simulink model "Cooperative_Quad_09_VelEst_02"  (R2017b)
settings: Solver=ode45  StartTime=0.0  StopTime=120  RelTol=1e-3  EnableMultiTasking=on
InitFcn:
  | Const_Vel_Est_02
values from neighbouring files (symbols this model uses):
  alpha = 1.0e-5    (= 1e-05)    [Cons_AMFC_Quad_New_01.m]    (also in Const_Vel_Est_02.m = 0.1; constant_Rev01_4Agents_10.m = 0.1; constant_Rev01_4Agents_9.m = 0.1)
  alpha_Slid = 0.01    [Cons_AMFC_Quad_New_01.m]    (also in Const_Vel_Est_02.m)
  AN = [     0 1 0 0 ... (first row only)    [Const_Vel_Est_02.m]    (also in constant_Rev01_4Agents_10.m; constant_Rev01_4Agents_9.m)
  B = 1e+0*eye(n)    [Cons_AMFC_Quad_New_01.m]    (also in Const_Vel_Est_02.m = 1e0*eye(n); constant_Rev01_4Agents_10.m = 1e0*eye(n); constant_Rev01_4Agents_9.m = 1e0*eye(n))
  BBT_inv = ((B'*B)^(-1))*B'    [Cons_AMFC_Quad_New_01.m]    (also in Const_Vel_Est_02.m; constant_Rev01_4Agents_10.m; constant_Rev01_4Agents_9.m)
  BN = [     1 0 0 0 ... (first row only)    [Const_Vel_Est_02.m]    (also in constant_Rev01_4Agents_10.m; constant_Rev01_4Agents_9.m)
  epsilon_struct = struct('data',epsilon_InitVal)    [Const_Vel_Est_02.m]    (also in constant_Rev01_4Agents_10.m; constant_Rev01_4Agents_9.m)
  g = 9.81    [Const_Vel_Est_02.m]    (also in Swing2d_01_const.m; constant_Rev01_4Agents_10.m; constant_Rev01_4Agents_9.m)
  gamma_0 = 1e-0*diag([1e-3*ones(3,1);1e-0*ones(3,1)])    [Cons_AMFC_Quad_New_01.m]    (also in Const_Vel_Est_02.m = 1e-1*diag([1e-3*ones(3,1);1e-0*ones(3,1)]); constant_Rev01_4Agents_10.m = 1e+1*diag([1e-3*ones(3,1);1e-0*ones(3,1)]); constant_Rev01_4Agents_9.m = 1e+1*diag([1e-3*ones(6,1);1e-0*ones(6,1)]))
  gamma_1 = 1e+2*diag([1e-3*ones(3,1);1e-0*ones(3,1)])    [Cons_AMFC_Quad_New_01.m]    (also in Const_Vel_Est_02.m; constant_Rev01_4Agents_10.m = 1e+3*diag([1e-3*ones(3,1);1e0*ones(3,1)]); constant_Rev01_4Agents_9.m = 1e+3*diag([1e-3*ones(6,1);1e0*ones(6,1)]))
  H = L + BN    [Const_Vel_Est_02.m]    (also in constant_Rev01_4Agents_10.m; constant_Rev01_4Agents_9.m)
  J = 1.2416e-3 * diag([1 1 2])    [Cons_AMFC_Quad_New_01.m]    (also in Const_Vel_Est_02.m = 1.2416e-3 * diag([1 1 2],0); constant_Rev01_4Agents_10.m = 1.2416e-3 * diag([1 1 2],0); constant_Rev01_4Agents_9.m = 1.2416e-3 * diag([1 1 2],0))
  k1 = 10    [Cons_AMFC_Quad_New_01.m]    (also in Const_Vel_Est_02.m = 1; constant_Rev01_4Agents_10.m = 1; constant_Rev01_4Agents_9.m = 1)
  k1o = 1000    [Cons_AMFC_Quad_New_01.m]    (also in Const_Vel_Est_02.m)
  k2 = 0.1    [Cons_AMFC_Quad_New_01.m]    (also in Const_Vel_Est_02.m; constant_Rev01_4Agents_10.m = 1; constant_Rev01_4Agents_9.m = 1)
  k2o = 100    [Cons_AMFC_Quad_New_01.m]    (also in Const_Vel_Est_02.m)
  Ka = 0.01    [Cons_AMFC_Quad_New_01.m]    (also in Const_Vel_Est_02.m; constant_Rev01_4Agents_10.m; constant_Rev01_4Agents_9.m)
  Kd = 0.01    [Cons_AMFC_Quad_New_01.m]    (also in Const_Vel_Est_02.m; constant_Rev01_4Agents_10.m; constant_Rev01_4Agents_9.m)
  Kf = 1.0e-5    (= 1e-05)    [Cons_AMFC_Quad_New_01.m]    (also in Const_Vel_Est_02.m; constant_Rev01_4Agents_10.m; constant_Rev01_4Agents_9.m)
  Kt = 0.0435 * Kf    (= 4.35e-07)    [Cons_AMFC_Quad_New_01.m]    (also in Const_Vel_Est_02.m = 1e-07; constant_Rev01_4Agents_10.m = 1e-07; constant_Rev01_4Agents_9.m = 1e-07)
  Lq = 0.2    [Const_Vel_Est_02.m]    (also in constant_Rev01_4Agents_10.m; constant_Rev01_4Agents_9.m)
  m = 6    [Cons_AMFC_Quad_New_01.m]    (also in Const_Vel_Est_02.m; Swing2d_01_const.m = 1)
  M = 2.95    [Cons_AMFC_Quad_New_01.m]    (also in Const_Vel_Est_02.m = 2; constant_Rev01_4Agents_10.m = 2; constant_Rev01_4Agents_9.m = 2)
  Mb_P = Mb_val_P*ones(np,1)    [Const_Vel_Est_02.m]
  Mb_V = Mb_val_V*ones(np,1)    [Const_Vel_Est_02.m]
  Mu_P = 10    [Const_Vel_Est_02.m]
  Mu_V = 10    [Const_Vel_Est_02.m]
  n = 6    [Cons_AMFC_Quad_New_01.m]    (also in Const_Vel_Est_02.m; constant_Rev01_4Agents_10.m; constant_Rev01_4Agents_9.m = 12)
  N = 4    [Const_Vel_Est_02.m]    (also in constant_Rev01_4Agents_10.m; constant_Rev01_4Agents_9.m)
  n0 = 3    [Const_Vel_Est_02.m]    (also in constant_Rev01_4Agents_10.m; constant_Rev01_4Agents_9.m)
  np = 2    [Const_Vel_Est_02.m]
  Observer_Gain = 100    [Const_Vel_Est_02.m]    (also in constant_Rev01_4Agents_10.m; constant_Rev01_4Agents_9.m)
  Observer_Gain1 = 100    [Const_Vel_Est_02.m]    (also in constant_Rev01_4Agents_10.m = 10; constant_Rev01_4Agents_9.m = 10)
  Q = 1e-1*eye(n)    [Cons_AMFC_Quad_New_01.m]    (also in Const_Vel_Est_02.m = 1e-2*eye(n); constant_Rev01_4Agents_10.m = 1e-3*eye(n); constant_Rev01_4Agents_9.m = 1e-3*eye(n))
  R = 1e+0*eye(m)    [Cons_AMFC_Quad_New_01.m]    (also in Const_Vel_Est_02.m = 1e-0*eye(n); constant_Rev01_4Agents_10.m = 1e-0*eye(n); constant_Rev01_4Agents_9.m = 1e-0*eye(n))
  rho_0 = 1e-1    (= 0.1)    [Cons_AMFC_Quad_New_01.m]    (also in Const_Vel_Est_02.m; constant_Rev01_4Agents_10.m = 10; constant_Rev01_4Agents_9.m = 10)
  rho_1 = 1e-0    (= 1)    [Cons_AMFC_Quad_New_01.m]    (also in Const_Vel_Est_02.m; constant_Rev01_4Agents_10.m = 0.1; constant_Rev01_4Agents_9.m = 0.1)
  T_struct = struct('data',T_InitVal)    [Const_Vel_Est_02.m]    (also in constant_Rev01_4Agents_10.m; constant_Rev01_4Agents_9.m)
  U_dot0_M = U_dot0_m*ones(n0,1)    [Const_Vel_Est_02.m]    (also in constant_Rev01_4Agents_10.m; constant_Rev01_4Agents_9.m)
  Upsilon_M = Upsilon_m*ones(n0,1)    [Const_Vel_Est_02.m]    (also in constant_Rev01_4Agents_10.m; constant_Rev01_4Agents_9.m)
undefined symbols (not defined in the file or in its folder): sigbuilder_block
(part 5 of 5)

== matlab function Cooperative_Quad_09_VelEst_02/Agent #4/Decenteralized Cooperaive Controller #4/Ali-4/Translational-4/Differentiator/Sliding differentiator1 ==
  data: Du1 output; e input; n parameter; k2 parameter
function Du1 = fcn(e,n,k2)

a=k2;

ABS = zeros(n,1);
for i=1:n
    if e(i)>0
        ABS(i) = e(i);
    else
        ABS(i) = -e(i);
    end
end
SGN = e ./ (ABS + 0.01);

Du1 = - a*SGN;

end

== matlab function Cooperative_Quad_09_VelEst_02/Agent #4/Decenteralized Cooperaive Controller #4/Ali-4/Translational-4/g-Estimator ==
  data: sigma input; g_hat input; P input; rho_1 parameter; gamma_1 parameter; Dg_hat output
function Dg_hat = fcn(sigma,g_hat,P,rho_1,gamma_1)

Dg_hat = - gamma_1 * P * sigma - rho_1 * gamma_1 * g_hat;

end

== matlab function Cooperative_Quad_09_VelEst_02/Agent #4/Decenteralized Cooperaive Controller #4/Ali-4/Translational-4/main ==
  data: sigma input; zeta input; u output; Dy_d input; R parameter; P input; a_hat input; B parameter; g_hat input; x input; Q parameter; BBT_inv parameter; n parameter
function u = fcn(sigma,zeta,Dy_d,R,P,a_hat,B,g_hat,x,Q,BBT_inv,n)

u1 = (1/2) * R * B' * P * sigma;
u2 = BBT_inv * (Dy_d - a_hat*x + (eye(n) + 2*(((P)^(-1)*Q)) + a_hat)*sigma - g_hat - zeta) - (3/4) * R * B' * P * sigma;

u = u1 + u2;

end

== matlab function Cooperative_Quad_09_VelEst_02/Agent #4/Decenteralized Cooperaive Controller #4/Ali-4/Translational-4/variable change ==
  data: X input; Xd input; x_mod output; u input; xd_mod output; e_mod output
function [x_mod,xd_mod,e_mod] = fcn(X,Xd,u)

x_mod = [X(1:3);X(7:9)];

xd_mod = [Xd;u(1:3)];

e_mod = xd_mod - x_mod;


end

== matlab function Cooperative_Quad_09_VelEst_02/Agent #4/Decenteralized Cooperaive Controller #4/Computing xd-4  ==
  data: q_i input; T_i input; xd output; Agent_Num input
function xd = fcn(q_i,T_i,Agent_Num)

xd = q_i + T_i(1,:)' + T_i(Agent_Num+1,:)';

end

== matlab function Cooperative_Quad_09_VelEst_02/Agent #4/Decenteralized Cooperaive Controller #4/Cooperative Observers for X-4/Differentiator2/Sliding differentiator ==
  data: u output; u1 input; e input; k1o parameter; alpha_Slid parameter
function u = fcn(u1,e,k1o,alpha_Slid)

b=k1o;

ABS = abs(e);
SGN = e ./ (ABS + alpha_Slid);
u = u1 - b*((ABS.^0.5).*SGN); 

end

== matlab function Cooperative_Quad_09_VelEst_02/Agent #4/Decenteralized Cooperaive Controller #4/Cooperative Observers for X-4/Differentiator2/Sliding differentiator1 ==
  data: Du1 output; e input; k2o parameter; alpha_Slid parameter
function Du1 = fcn(e,k2o,alpha_Slid)

a=k2o;

ABS = abs(e);
SGN = e ./ (ABS + alpha_Slid);
Du1 = - a*SGN;

end

== matlab function Cooperative_Quad_09_VelEst_02/Agent #4/Decenteralized Cooperaive Controller #4/Cooperative Observers for X-4/MATLAB Function ==
  data: X_inp input; X_est output; P_est_XY input; Pos_local_Z input; V_est_XY input; V_local_Z input
function X_est = fcn(X_inp,P_est_XY,Pos_local_Z,V_est_XY,V_local_Z)

X_est = [P_est_XY;Pos_local_Z;X_inp(4:6);V_est_XY;V_local_Z;X_inp(10:12)];

end

== matlab function Cooperative_Quad_09_VelEst_02/Agent #4/Decenteralized Cooperaive Controller #4/Cooperative Observers for X-4/Pos observer-4 ==
  data: P_hat input; tau input; P0 input; P_rel_local input; P_rel0_local input; AN parameter; BN parameter; H parameter; DP_hat_local output; np parameter; N parameter; Num input; Mu_P parameter; Mb_P parameter; tau_i output; alpha parameter
function [DP_hat_local,tau_i] = fcn(P_hat,tau,P0,P_rel_local,P_rel0_local,AN,BN,H,np,N,Num,Mu_P,Mb_P,alpha)

P_hat_in = zeros(np,N);
P_rel_local_in = zeros(np,N);
tau_in = zeros(np,N);
for i=1:N
    P_hat_in(:,i) = P_hat((i-1)*np+1:(i*np),1); 
    P_rel_local_in(:,i) = P_rel_local((i-1)*np+1:(i*np),1); 
    tau_in(:,i) = tau((i-1)*np+1:(i*np),1);
end

e = BN(Num,Num)*(P_hat_in(:,Num) - (P0 + P_rel0_local));
Vec = zeros(np,1);
for i=1:N
    e = e + ( AN(Num,i)*(P_hat_in(:,Num) - (P_hat_in(:,i) + P_rel_local_in(:,i))) ); 
    Vec = Vec + ( H(Num,i)*tau_in(:,i) );    
end

SGN_vec = Vec./(abs(Vec)+alpha);
SGN = diag(SGN_vec);    

DP_hat_local = - ( Mu_P*e ) - ( SGN*Mb_P );
tau_i = e;

end

== matlab function Cooperative_Quad_09_VelEst_02/Agent #4/Decenteralized Cooperaive Controller #4/Cooperative Observers for X-4/Vel observer-4 ==
  data: P_hat input; tau input; P0 input; P_rel_local input; P_rel0_local input; AN parameter; BN parameter; H parameter; DP_hat_local output; np parameter; N parameter; Num input; Mu_V parameter; Mb_V parameter; tau_i output; alpha parameter
function [DP_hat_local,tau_i] = fcn(P_hat,tau,P0,P_rel_local,P_rel0_local,AN,BN,H,np,N,Num,Mu_V,Mb_V,alpha)

P_hat_in = zeros(np,N);
P_rel_local_in = zeros(np,N);
tau_in = zeros(np,N);
for i=1:N
    P_hat_in(:,i) = P_hat((i-1)*np+1:(i*np),1); 
    P_rel_local_in(:,i) = P_rel_local((i-1)*np+1:(i*np),1); 
    tau_in(:,i) = tau((i-1)*np+1:(i*np),1);
end

e = BN(Num,Num)*(P_hat_in(:,Num) - (P0 + P_rel0_local));
Vec = zeros(np,1);
for i=1:N
    e = e + ( AN(Num,i)*(P_hat_in(:,Num) - (P_hat_in(:,i) + P_rel_local_in(:,i))) ); 
    Vec = Vec + ( H(Num,i)*tau_in(:,i) );    
end

SGN_vec = Vec./(abs(Vec)+alpha);
SGN = diag(SGN_vec);    

DP_hat_local = - ( Mu_V*e ) - ( SGN*Mb_V );
tau_i = e;

end

== matlab function Cooperative_Quad_09_VelEst_02/Agent #4/Decenteralized Cooperaive Controller #4/Cooperative Observers for Xd-4/Observer T#4 ==
  data: T_struct parameter; T input; DT_i output; epsilon input; epsilon_struct parameter; H parameter; BN parameter; AN parameter; T_i input; chi input; Upsilon_M parameter; epsilon_i output; N parameter; n0 parameter; Agent_Num input; Observer_Gain1 parameter; alpha parameter
function [DT_i,epsilon_i] = fcn(T_struct,T,epsilon,epsilon_struct,H,BN,AN,T_i,chi,Upsilon_M,N,n0,...
    Agent_Num,Observer_Gain1,alpha)

T_struct(1).data = T.t1;
T_struct(2).data = T.t2;
T_struct(3).data = T.t3;
T_struct(4).data = T.t4;

epsilon_struct(1).data = epsilon.eps1;
epsilon_struct(2).data = epsilon.eps2;
epsilon_struct(3).data = epsilon.eps3;
epsilon_struct(4).data = epsilon.eps4;

epsilon_i = + BN(Agent_Num,Agent_Num)*(T_i - chi);
Sum2 = zeros(N+1,n0);
for i=1:N
    epsilon_i = epsilon_i + ( AN(Agent_Num,i) * (T_i - T_struct(i).data) );  
    Sum2 = Sum2 + ( H(i,Agent_Num) * epsilon_struct(i).data );
end

Sum21 = abs(Sum2) + alpha;
SGN2 = Sum2./Sum21;

DT_i = -Observer_Gain1*epsilon_i - SGN2*diag(Upsilon_M);

end

== matlab function Cooperative_Quad_09_VelEst_02/Agent #4/Decenteralized Cooperaive Controller #4/Cooperative Observers for Xd-4/Observer q#4 ==
  data: q input; Dq_i output; tau input; H parameter; BN parameter; AN parameter; q_i input; u0 input; U_dot0_M parameter; tau_i output; N parameter; Agent_Num input; Observer_Gain parameter; n0 parameter; alpha parameter
function [Dq_i,tau_i] = fcn(q,tau,H,BN,AN,q_i,u0,U_dot0_M,N,Agent_Num,Observer_Gain,n0,alpha)

tau_i = + BN(Agent_Num,Agent_Num)*(q_i - u0);
Sum2 = zeros(n0,1);
for i=1:N
    tau_i = tau_i + ( AN(Agent_Num,i) * (q_i - q(((i-1)*n0+1):n0*i)) );  
    Sum2 = Sum2 + ( H(i,Agent_Num) * tau(((i-1)*n0+1):n0*i) );
end

Sum21 = abs(Sum2) + alpha;
SGN2 = Sum2./Sum21;

Dq_i = -Observer_Gain*tau_i - diag(SGN2)*U_dot0_M;

end

== matlab function Cooperative_Quad_09_VelEst_02/Agent #4/Plant #4/MATLAB Function ==
  data: X input; u1 input; u2 input; u3 input; u4 input; t input; DX output; Kf parameter; Kt parameter; Kd parameter; Ka parameter; M parameter; J parameter; Lq parameter; g parameter; Pos_XY output; Pos_Z output; Vel_XY output; Acc_XY output
function [DX,Pos_XY,Pos_Z,Vel_XY,Acc_XY] = fcn(X,u1,u2,u3,u4,t,Kf,Kt,Kd,Ka,M,J,Lq,g)

F1 = Kf * u1^2;
F2 = Kf * u2^2;
F3 = Kf * u3^2;
F4 = Kf * u4^2;
 
FT = F1 + F2 + F3 + F4;

T1 = Kt * u1^2;
T2 = Kt * u2^2;
T3 = Kt * u3^2;
T4 = Kt * u4^2;

phi = X(4);
theta = X(5);
psi = X(6);

Rq = [cos(psi)*cos(theta) -sin(psi)*cos(phi)+cos(psi)*sin(theta)*sin(phi) sin(psi)*sin(phi)+cos(psi)*sin(theta)*cos(phi);
    sin(psi)*cos(theta) cos(psi)*cos(phi)+sin(psi)*sin(theta)*sin(phi) -cos(psi)*sin(phi)+sin(psi)*sin(theta)*cos(phi);
    -sin(theta) cos(theta)*sin(phi) cos(theta)*cos(phi)]; 

R_omega = [1 0 -sin(theta);
    0 cos(phi) cos(theta)*sin(phi);
    0 -sin(phi) cos(theta)*cos(phi)];

EXT_PRD = External_Product3(X(10:12),(J*X(10:12)));

DP = X(7:9);
DPHI = R_omega^(-1) * X(10:12); 
Dv = (1/M)*(Rq*[0;0;FT] - Kd*X(7:9) - M*[0;0;g]) + Rq*(1*sin(1*t))*[0;0;1];
Dw = (J^(-1))*([Lq*(F3-F1);Lq*(F4-F2);(T1-T2+T3-T4)] - Ka*X(10:12) - EXT_PRD) + (1*sin(1*t));

DX = [DP;DPHI;Dv;Dw];

Pos_XY = X(1:2);
Pos_Z = X(3);
Vel_XY = X(7:8);
Acc_XY = DX(7:8);

end

== matlab function Cooperative_Quad_09_VelEst_02/Agent #4/Relative estimations-4/Rel_40/Differentiator1/Sliding differentiator ==
  data: u output; u1 input; e input; k1o parameter; alpha_Slid parameter
function u = fcn(u1,e,k1o,alpha_Slid)

b=k1o;

ABS = abs(e);
SGN = e ./ (ABS + alpha_Slid);
u = u1 - b*((ABS.^0.5).*SGN); 

end

== matlab function Cooperative_Quad_09_VelEst_02/Agent #4/Relative estimations-4/Rel_40/Differentiator1/Sliding differentiator1 ==
  data: Du1 output; e input; k2o parameter; alpha_Slid parameter
function Du1 = fcn(e,k2o,alpha_Slid)

a=k2o;

ABS = abs(e);
SGN = e ./ (ABS + alpha_Slid);
Du1 = - a*SGN;

end

== matlab function Cooperative_Quad_09_VelEst_02/Agent #4/Relative estimations-4/Rel_40/Relative estimation1 ==
  data: V_rel input; dp input; DP_est output; P_est input; alpha_P parameter
function DP_est = fcn(V_rel,dp,P_est,alpha_P)

ep = (dp^2) - (P_est'*P_est);
gp = P_est'*V_rel;

DP_est = (1 + alpha_P * sign(ep*gp)) * V_rel;

end

== matlab function Cooperative_Quad_09_VelEst_02/Agent #4/Relative estimations-4/Rel_40/Relative estimation2 ==
  data: A_rel input; dv input; DV_est output size=2; V_est input size=2; alpha_V parameter
function DV_est = fcn(A_rel,dv,V_est,alpha_V)

ev = (dv^2) - (V_est'*V_est);
gv = V_est'*A_rel;

DV_est = (1 + alpha_V * sign(ev*gv)) * A_rel;

end

== matlab function Cooperative_Quad_09_VelEst_02/Agent #4/Relative estimations-4/Rel_40/Relative measurements1 ==
  data: P_other input; d output; P_local input
function d = fcn(P_other,P_local)

P2 = P_local;
P1 = P_other;

d = sqrt( (P2(1) - P1(1))^2 + (P2(2) - P1(2))^2 );

end

== matlab function Cooperative_Quad_09_VelEst_02/Agent #4/Relative estimations-4/Rel_41/Differentiator1/Sliding differentiator ==
  data: u output; u1 input; e input; k1o parameter; alpha_Slid parameter
function u = fcn(u1,e,k1o,alpha_Slid)

b=k1o;

ABS = abs(e);
SGN = e ./ (ABS + alpha_Slid);
u = u1 - b*((ABS.^0.5).*SGN); 

end

== matlab function Cooperative_Quad_09_VelEst_02/Agent #4/Relative estimations-4/Rel_41/Differentiator1/Sliding differentiator1 ==
  data: Du1 output; e input; k2o parameter; alpha_Slid parameter
function Du1 = fcn(e,k2o,alpha_Slid)

a=k2o;

ABS = abs(e);
SGN = e ./ (ABS + alpha_Slid);
Du1 = - a*SGN;

end

== matlab function Cooperative_Quad_09_VelEst_02/Agent #4/Relative estimations-4/Rel_41/Relative estimation1-2 ==
  data: A_rel input; dv input; DV_est output size=2; V_est input size=2; alpha_V parameter
function DV_est = fcn(A_rel,dv,V_est,alpha_V)

ev = (dv^2) - (V_est'*V_est);
gv = V_est'*A_rel;

DV_est = (1 + alpha_V * sign(ev*gv)) * A_rel;

end

== matlab function Cooperative_Quad_09_VelEst_02/Agent #4/Relative estimations-4/Rel_41/Relative estimation2 ==
  data: V_rel input; dp input; DP_est output; P_est input; alpha_P parameter
function DP_est = fcn(V_rel,dp,P_est,alpha_P)

ep = (dp^2) - (P_est'*P_est);
gp = P_est'*V_rel;

DP_est = (1 + alpha_P * sign(ep*gp)) * V_rel;

end

== matlab function Cooperative_Quad_09_VelEst_02/Agent #4/Relative estimations-4/Rel_41/Relative measurements2 ==
  data: P_other input; d output; P_local input
function d = fcn(P_other,P_local)

P2 = P_local;
P1 = P_other;

d = sqrt( (P2(1) - P1(1))^2 + (P2(2) - P1(2))^2 );

end

== matlab function Cooperative_Quad_09_VelEst_02/Agent #4/Relative estimations-4/Rel_42/Differentiator1/Sliding differentiator ==
  data: u output; u1 input; e input; k1o parameter; alpha_Slid parameter
function u = fcn(u1,e,k1o,alpha_Slid)

b=k1o;

ABS = abs(e);
SGN = e ./ (ABS + alpha_Slid);
u = u1 - b*((ABS.^0.5).*SGN); 

end

== matlab function Cooperative_Quad_09_VelEst_02/Agent #4/Relative estimations-4/Rel_42/Differentiator1/Sliding differentiator1 ==
  data: Du1 output; e input; k2o parameter; alpha_Slid parameter
function Du1 = fcn(e,k2o,alpha_Slid)

a=k2o;

ABS = abs(e);
SGN = e ./ (ABS + alpha_Slid);
Du1 = - a*SGN;

end

== matlab function Cooperative_Quad_09_VelEst_02/Agent #4/Relative estimations-4/Rel_42/Relative estimation1-2 ==
  data: A_rel input; dv input; DV_est output size=2; V_est input size=2; alpha_V parameter
function DV_est = fcn(A_rel,dv,V_est,alpha_V)

ev = (dv^2) - (V_est'*V_est);
gv = V_est'*A_rel;

DV_est = (1 + alpha_V * sign(ev*gv)) * A_rel;

end

== matlab function Cooperative_Quad_09_VelEst_02/Agent #4/Relative estimations-4/Rel_42/Relative estimation2 ==
  data: V_rel input; dp input; DP_est output; P_est input; alpha_P parameter
function DP_est = fcn(V_rel,dp,P_est,alpha_P)

ep = (dp^2) - (P_est'*P_est);
gp = P_est'*V_rel;

DP_est = (1 + alpha_P * sign(ep*gp)) * V_rel;

end

== matlab function Cooperative_Quad_09_VelEst_02/Agent #4/Relative estimations-4/Rel_42/Relative measurements2 ==
  data: P_other input; d output; P_local input
function d = fcn(P_other,P_local)

P2 = P_local;
P1 = P_other;

d = sqrt( (P2(1) - P1(1))^2 + (P2(2) - P1(2))^2 );

end

== matlab function Cooperative_Quad_09_VelEst_02/Agent #4/Relative estimations-4/Rel_43/Differentiator1/Sliding differentiator ==
  data: u output; u1 input; e input; k1o parameter; alpha_Slid parameter
function u = fcn(u1,e,k1o,alpha_Slid)

b=k1o;

ABS = abs(e);
SGN = e ./ (ABS + alpha_Slid);
u = u1 - b*((ABS.^0.5).*SGN); 

end

== matlab function Cooperative_Quad_09_VelEst_02/Agent #4/Relative estimations-4/Rel_43/Differentiator1/Sliding differentiator1 ==
  data: Du1 output; e input; k2o parameter; alpha_Slid parameter
function Du1 = fcn(e,k2o,alpha_Slid)

a=k2o;

ABS = abs(e);
SGN = e ./ (ABS + alpha_Slid);
Du1 = - a*SGN;

end

== matlab function Cooperative_Quad_09_VelEst_02/Agent #4/Relative estimations-4/Rel_43/Relative estimation1 ==
  data: V_rel input; dp input; DP_est output; P_est input; alpha_P parameter
function DP_est = fcn(V_rel,dp,P_est,alpha_P)

ep = (dp^2) - (P_est'*P_est);
gp = P_est'*V_rel;

DP_est = (1 + alpha_P * sign(ep*gp)) * V_rel;

end

== matlab function Cooperative_Quad_09_VelEst_02/Agent #4/Relative estimations-4/Rel_43/Relative estimation2 ==
  data: A_rel input; dv input; DV_est output size=2; V_est input size=2; alpha_V parameter
function DV_est = fcn(A_rel,dv,V_est,alpha_V)

ev = (dv^2) - (V_est'*V_est);
gv = V_est'*A_rel;

DV_est = (1 + alpha_V * sign(ev*gv)) * A_rel;

end

== matlab function Cooperative_Quad_09_VelEst_02/Agent #4/Relative estimations-4/Rel_43/Relative measurements1 ==
  data: P_other input; d output; P_local input
function d = fcn(P_other,P_local)

P2 = P_local;
P1 = P_other;

d = sqrt( (P2(1) - P1(1))^2 + (P2(2) - P1(2))^2 );

end

== matlab function Cooperative_Quad_09_VelEst_02/Data Bus /Communications for controllers/For matrix Plot16/MATLAB Function ==
  data: u input; y output
function y = fcn(u)
S1 = size(u,1);
S2 = size(u,2);

y = zeros(S1*S2,1);
num = 0;
for i=1:S1
    for j=1:S2
        num = num + 1;
        y(num,1) = u(i,j);
    end
end

end

== matlab function Cooperative_Quad_09_VelEst_02/Data Bus /Communications for controllers/For matrix Plot17/MATLAB Function ==
  data: u input; y output
function y = fcn(u)
S1 = size(u,1);
S2 = size(u,2);

y = zeros(S1*S2,1);
num = 0;
for i=1:S1
    for j=1:S2
        num = num + 1;
        y(num,1) = u(i,j);
    end
end

end

== matlab function Cooperative_Quad_09_VelEst_02/Data Bus /Communications for controllers/For matrix Plot18/MATLAB Function ==
  data: u input; y output
function y = fcn(u)
S1 = size(u,1);
S2 = size(u,2);

y = zeros(S1*S2,1);
num = 0;
for i=1:S1
    for j=1:S2
        num = num + 1;
        y(num,1) = u(i,j);
    end
end

end

== matlab function Cooperative_Quad_09_VelEst_02/Data Bus /Communications for controllers/For matrix Plot19/MATLAB Function ==
  data: u input; y output
function y = fcn(u)
S1 = size(u,1);
S2 = size(u,2);

y = zeros(S1*S2,1);
num = 0;
for i=1:S1
    for j=1:S2
        num = num + 1;
        y(num,1) = u(i,j);
    end
end

end

== matlab function Cooperative_Quad_09_VelEst_02/Data Bus /Communications for controllers/For matrix Plot20/MATLAB Function ==
  data: u input; y output
function y = fcn(u)
S1 = size(u,1);
S2 = size(u,2);

y = zeros(S1*S2,1);
num = 0;
for i=1:S1
    for j=1:S2
        num = num + 1;
        y(num,1) = u(i,j);
    end
end

end

== matlab function Cooperative_Quad_09_VelEst_02/Data Bus /Communications for controllers/For matrix Plot21/MATLAB Function ==
  data: u input; y output
function y = fcn(u)
S1 = size(u,1);
S2 = size(u,2);

y = zeros(S1*S2,1);
num = 0;
for i=1:S1
    for j=1:S2
        num = num + 1;
        y(num,1) = u(i,j);
    end
end

end

== matlab function Cooperative_Quad_09_VelEst_02/Data Bus /Communications for controllers/For matrix Plot22/MATLAB Function ==
  data: u input; y output
function y = fcn(u)
S1 = size(u,1);
S2 = size(u,2);

y = zeros(S1*S2,1);
num = 0;
for i=1:S1
    for j=1:S2
        num = num + 1;
        y(num,1) = u(i,j);
    end
end

end

== matlab function Cooperative_Quad_09_VelEst_02/Data Bus /Communications for controllers/For matrix Plot23/MATLAB Function ==
  data: u input; y output
function y = fcn(u)
S1 = size(u,1);
S2 = size(u,2);

y = zeros(S1*S2,1);
num = 0;
for i=1:S1
    for j=1:S2
        num = num + 1;
        y(num,1) = u(i,j);
    end
end

end

== matlab function Cooperative_Quad_09_VelEst_02/Data Bus /Reference Trajectory/Differentiator/Sliding differentiator ==
  data: u output; u1 input; e input; np parameter; k1 parameter
function u = fcn(u1,e,np,k1)

b=k1;

ABS = zeros(np,1);
for i=1:np
    if e(i)>0
        ABS(i) = e(i);
    else
        ABS(i) = -e(i);
    end
end
SGN = e ./ (ABS + 0.01);

u = u1 - b*(ABS.^0.5).*SGN;

end

== matlab function Cooperative_Quad_09_VelEst_02/Data Bus /Reference Trajectory/Differentiator/Sliding differentiator1 ==
  data: Du1 output; e input; np parameter; k2 parameter
function Du1 = fcn(e,np,k2)

a=k2;

ABS = zeros(np,1);
for i=1:np
    if e(i)>0
        ABS(i) = e(i);
    else
        ABS(i) = -e(i);
    end
end
SGN = e ./ (ABS + 0.01);

Du1 = - a*SGN;

end

== matlab function Cooperative_Quad_09_VelEst_02/Data Bus /Reference Trajectory/Differentiator1/Sliding differentiator ==
  data: u output; u1 input; e input; np parameter; k1 parameter
function u = fcn(u1,e,np,k1)

b=k1;

ABS = zeros(np,1);
for i=1:np
    if e(i)>0
        ABS(i) = e(i);
    else
        ABS(i) = -e(i);
    end
end
SGN = e ./ (ABS + 0.01);

u = u1 - b*(ABS.^0.5).*SGN;

end

== matlab function Cooperative_Quad_09_VelEst_02/Data Bus /Reference Trajectory/Differentiator1/Sliding differentiator1 ==
  data: Du1 output; e input; np parameter; k2 parameter
function Du1 = fcn(e,np,k2)

a=k2;

ABS = zeros(np,1);
for i=1:np
    if e(i)>0
        ABS(i) = e(i);
    else
        ABS(i) = -e(i);
    end
end
SGN = e ./ (ABS + 0.01);

Du1 = - a*SGN;

end
